simulink model "controller_for_bicycleROS"  (R2021a)
settings: Solver=VariableStepAuto  StartTime=0.0  StopTime=10.0  RelTol=1e-3
values from neighbouring files (symbols this model uses):
  Fyf = zeros(1,57)    [FyfLookUpNewCar.m]    (also in Fyf_loopup_table.mat = [-9372.31873381 -9371.87234491 -9368.75632133 -9360.32413915)
  SlipAngle = -SlipAngle    [FyfLookUpNewCar.m]    (also in Fyf_loopup_table.mat = [0.153111393254 0.147643129209 0.142174865164 0.13670660112 )
  Vx = 15    [controller_setup.m]
libraries: robotlib x22, simulink_extras x1, autolibshared x1, simulink x1
settings Model: Creator=chnwa  LastModifiedBy=chnwa

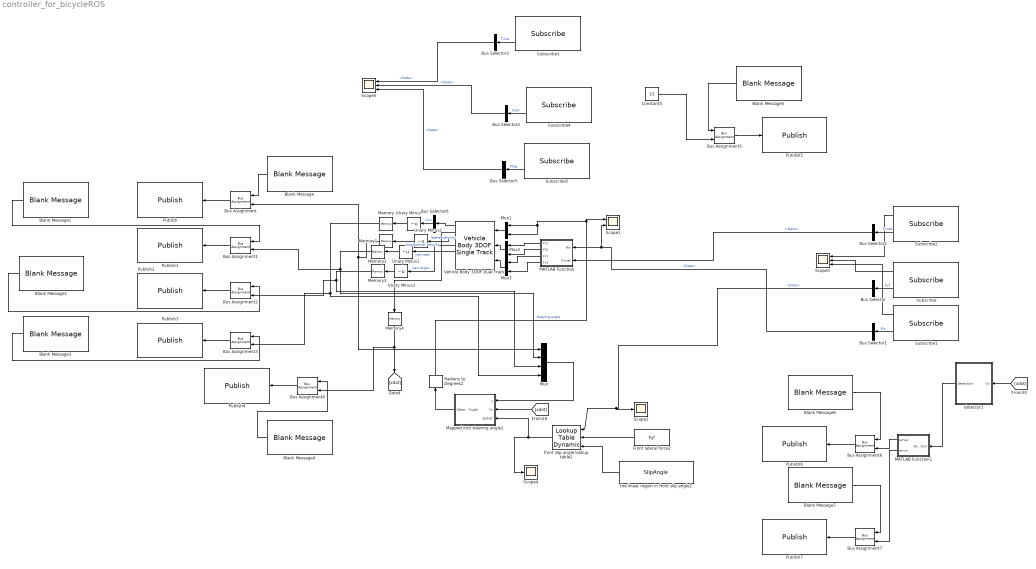
== system controller_for_bicycleROS ==
  Blank Message{,1..7} (8 alike) : robotlib/Blank Message  messageClass=Message  entityType=std_msgs/Float64  messageType=std_msgs/Float64  SampleTime=inf  legacyBusStruct=off
  Bus Assignment{,1..7} (8 alike) : BusAssignment  AssignedSignals=Data
  Bus Selector{,1..5} (6 alike) : BusSelector  OutputSignals=Data
  Bus Selector6 : BusSelector  OutputSignals=InertFrm.Cg.Disp.Y
  Constant5 : Constant  Value=15
  Front lateral force2 : Constant  Value=Fyf
  MATLAB Function : MATLAB Function  TreatAsAtomicUnit=on
  MATLAB Function1 : MATLAB Function  TreatAsAtomicUnit=on
  Mapped into steering angle2 : MATLAB Function  TreatAsAtomicUnit=on
  Memory{,1..3} (4 alike) : Memory
  Memory4 : Memory  InitialCondition=15
  Mux : Mux
  Mux1 : Mux  Inputs=2
  Mux2 : Mux  Inputs=2
  Mux3 : Mux  Inputs=2
  Publish : robotlib/Publish  topicSource=Specify your own  topic=/states1  messageType=std_msgs/Float64  legacyBusStruct=off  messageQueueLength=1
  Publish1 : robotlib/Publish  topicSource=Specify your own  topic=/states2  messageType=std_msgs/Float64  legacyBusStruct=off  messageQueueLength=1
  Publish2 : robotlib/Publish  topicSource=Specify your own  topic=/states3  messageType=std_msgs/Float64  legacyBusStruct=off  messageQueueLength=1
  Publish3 : robotlib/Publish  topicSource=Specify your own  topic=/states4  messageType=std_msgs/Float64  legacyBusStruct=off  messageQueueLength=1
  Publish4 : robotlib/Publish  topicSource=Specify your own  topic=/Vx  messageType=std_msgs/Float64  legacyBusStruct=off  messageQueueLength=1
  Publish5 : robotlib/Publish  topicSource=Specify your own  topic=/Vset  messageType=std_msgs/Float64  legacyBusStruct=off  messageQueueLength=1
  Publish6 : robotlib/Publish  topicSource=Specify your own  topic=/emax  messageType=std_msgs/Float64  legacyBusStruct=off  messageQueueLength=1
  Publish7 : robotlib/Publish  topicSource=Specify your own  topic=/emin  messageType=std_msgs/Float64  legacyBusStruct=off  messageQueueLength=1
  Radians to Degrees2 : simulink_extras/Transformations/Radians to Degrees
  Scope1 : Scope  NumInputPorts=2
  Scope2 : Scope
  Scope3 : Scope  NumInputPorts=3
  Scope4 : Scope
  Scope5 : Scope  NumInputPorts=3
  Subscribe : robotlib/Subscribe  topicSource=Specify your own  topic=/mv1  messageType=std_msgs/Float64  SampleTime=-1  legacyBusStruct=off  messageQueueLength=1
  Subscribe1 : robotlib/Subscribe  topicSource=Specify your own  topic=/mv2  messageType=std_msgs/Float64  SampleTime=-1  legacyBusStruct=off  messageQueueLength=1
  Subscribe2 : robotlib/Subscribe  topicSource=Specify your own  topic=/Fxnet  messageType=std_msgs/Float64  SampleTime=-1  legacyBusStruct=off  messageQueueLength=1
  Subscribe3 : robotlib/Subscribe  topicSource=Specify your own  topic=/Time  messageType=std_msgs/Float64  SampleTime=-1  legacyBusStruct=off  messageQueueLength=1
  Subscribe4 : robotlib/Subscribe  topicSource=Specify your own  topic=/Cost  messageType=std_msgs/Float64  SampleTime=-1  legacyBusStruct=off  messageQueueLength=1
  Subscribe5 : robotlib/Subscribe  topicSource=Specify your own  topic=/Flag  messageType=std_msgs/Float64  SampleTime=-1  legacyBusStruct=off  messageQueueLength=1
  Unary Minus{,1..3} (4 alike) : UnaryMinus
  Vehicle Body 3DOF Dual Track : autolibshared/Vehicle Body 3DOF Single Track  trackMode=Dual  inputMode=External longitudinal forces  frontSteerMode=on  rearSteerMode=off  windMode=off  muMode=off  extFMode=off  extMMode=off  htchFMode=off  htchMMode=off  extXo=off  extpsio=off  extxdoto=off  extro=off  extYo=off  extTamb=off  extydoto=off  aMode=2  NF=2  NR=2  m=2272  a=1.11  b=1.67  h=0.35  dh=1  hh=0.2  X_o=0  xdot_o=15  CalphaMode=off  sigmaMode=on  d=0  hl=0  w=[1.4,1.4]  Cy_f=1.822e5  Cy_r=1.822e5  sigma_f=.1  sigma_r=.1  alpha_f_brk=[-.1 .1]  Cy_f_data=[-9e3 9e3]  alpha_r_brk=[-.1 .1]  Cy_r_data=[-9e3 9e3]  Y_o=0  ydot_o=0  Izz=4600  psi_o=0  r_o=0  Af=2  Cd=.3  Cl=.1  Cpm=.1  beta_w=[0:0.01:0.3]  Cs=[0:0.03:0.9]  Cym=[0:0.01:0.3]  Pabs=101325  Tair=273  g=9.81  mu=0.7  xdot_tol=.01  Fznom=5000  Fxtire_sat=7e4  Fytire_sat=7e4  longOff=0  latOff=0  vertOff=0  wrapAng=off
      settings: SourceProductBaseCode=PW,DR,MT,UV,VE
  detector1 : Subsystem
  front slip angle lookup table2 : simulink/Lookup Tables/Lookup Table Dynamic  LookUpMeth=Interpolation-Use End Values  OutDataType=fixdt('double')  OutScaling=[]  OutputDataTypeScalingMode=Specify via dialog  OutDataTypeStr=double  DoSatur=off
  tire linear region in front slip angle2 : Constant  Value=SlipAngle
  wires:
  MATLAB Function/2(Fl2) -> Mux2/2
  Mapped into steering angle2/1(SteeringAngle) -> Radians to Degrees2/1
  Bus Selector4/1 -> Scope5/2  "<Data>"
  Constant5/1 -> Bus Assignment5/2
  Bus Assignment4/1 -> Publish4/1
  Bus Selector5/1 -> Scope5/3  "<Data>"
  Bus Selector3/1 -> Scope5/1  "<Data>"
  Vehicle Body 3DOF Dual Track/3 -> Unary Minus2/1  "lateral velocity"
  Bus Selector/1 -> Scope2/1, front slip angle lookup table2/1  "<Data>"
  Front lateral force2/1 -> front slip angle lookup table2/2
  detector1/1(detection) -> MATLAB Function1/1(detection)
  Blank Message2/1 -> Bus Assignment2/1
  Subscribe/2 -> Bus Selector/1  "Fyf"
  Bus Assignment7/1 -> Publish7/1
  Blank Message1/1 -> Bus Assignment1/1
  MATLAB Function/3(Fr1) -> Mux3/1
  Blank Message7/1 -> Bus Assignment7/1
  Blank Message6/1 -> Bus Assignment6/1
  Bus Assignment3/1 -> Publish3/1
  Bus Selector1/1 -> Scope1/2, MATLAB Function/1(Mx)  "<Data>"
  Subscribe5/2 -> Bus Selector5/1  "Flag"
  Bus Assignment2/1 -> Publish2/1
  Bus Assignment6/1 -> Publish6/1
  Vehicle Body 3DOF Dual Track/4 -> Unary Minus3/1  "yaw angle"
  Subscribe1/2 -> Bus Selector1/1  "Mx"
  Bus Assignment/1 -> Publish/1
  MATLAB Function1/1(emax) -> Bus Assignment6/2
  Bus Selector2/1 -> MATLAB Function/2(Fxnet)  "<Data>"
  Subscribe/1 -> Scope3/2
  Blank Message/1 -> Bus Assignment/1
  Subscribe1/1 -> Scope3/3
  Blank Message4/1 -> Bus Assignment4/1
  Radians to Degrees2/1 -> Mux1/2, Mux1/1, Scope1/1  "steering angle"
  Subscribe4/2 -> Bus Selector4/1  "Cost"
  Bus Assignment5/1 -> Publish5/1
  Subscribe3/2 -> Bus Selector3/1  "Time"
  front slip angle lookup table2/1 -> Scope4/1, Mapped into steering angle2/3(alphaf)
  MATLAB Function1/2(emin) -> Bus Assignment7/2
  MATLAB Function/4(Fr2) -> Mux3/2
  Bus Selector6/1 -> Unary Minus/1  "<Y>"
  MATLAB Function/1(Fl1) -> Mux2/1
  Blank Message5/1 -> Bus Assignment5/1
  Mux/1 -> Mapped into steering angle2/1(x)
  Bus Assignment1/1 -> Publish1/1
  Subscribe2/2 -> Bus Selector2/1  "Fxnet"
  Vehicle Body 3DOF Dual Track/5 -> Unary Minus1/1  "yaw rate"
  Blank Message3/1 -> Bus Assignment3/1
  Subscribe2/1 -> Scope3/1
  tire linear region in front slip angle2/1 -> front slip angle lookup table2/3
  [xdot] -> Mapped into steering angle2/2(Vx)
  [xdot] -> detector1/1(Vx)
  Vehicle Body 3DOF Dual Track/2 -> Memory4/1  "longitudinal velocity"
  Mux2/1 -> Vehicle Body 3DOF Dual Track/2
  Mux1/1 -> Vehicle Body 3DOF Dual Track/1
  Mux3/1 -> Vehicle Body 3DOF Dual Track/3
  Vehicle Body 3DOF Dual Track/1 -> Bus Selector6/1
  Unary Minus/1 -> Memory/1
  Unary Minus2/1 -> Memory1/1
  Unary Minus3/1 -> Memory3/1
  Unary Minus1/1 -> Memory2/1
  Memory/1 -> Mux/4, Bus Assignment3/2
  Memory1/1 -> Bus Assignment/2, Mux/1
  Memory2/1 -> Mux/2, Bus Assignment1/2
  Memory3/1 -> Mux/3, Bus Assignment2/2
  Memory4/1 -> [xdot], Bus Assignment4/2

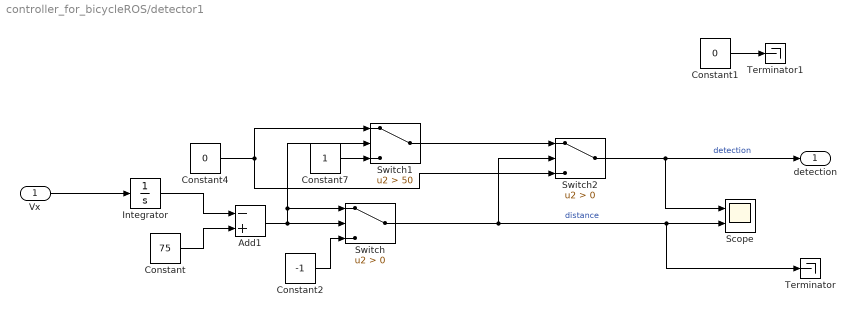
== system controller_for_bicycleROS/detector1 ==
  Vx : Inport
  Add1 : Sum  Inputs=-+
  Constant : Constant  Value=75
  Constant1 : Constant  Value=0
  Constant2 : Constant  Value=-1
  Constant4 : Constant  Value=0
  Constant7 : Constant
  Integrator : Integrator
  Scope : Scope  NumInputPorts=2
  Switch : Switch  Criteria=u2 > Threshold
  Switch1 : Switch  Criteria=u2 > Threshold  Threshold=50
  Switch2 : Switch  Criteria=u2 > Threshold
  Terminator : Terminator
  Terminator1 : Terminator
  detection : Outport
  wires:
  Constant2/1 -> Switch/3
  Constant4/1 -> Switch2/3, Switch1/1
  Vx/1 -> Integrator/1
  Integrator/1 -> Add1/1
  Switch/1 -> Switch2/2, Terminator/1, Scope/2  "distance"
  Constant7/1 -> Switch1/3
  Add1/1 -> Switch1/2, Switch/1, Switch/2
  Switch1/1 -> Switch2/1
  Constant/1 -> Add1/2
  Switch2/1 -> detection/1, Scope/1  "detection"
  Constant1/1 -> Terminator1/1

== matlab function controller_for_bicycleROS/MATLAB Function1 ==
  data: detection input; emax output; emin output
function [emax,emin] = fcn(detection)

if detection
    emax=6;
    emin=4;
else
    emax=10;
    emin=-10;
end

== matlab function controller_for_bicycleROS/Mapped into steering angle2 ==
  data: x input; Vx input; alphaf input; SteeringAngle output
function SteeringAngle = fcn(x,Vx, alphaf)

lf = 1.11;  % distance from front axle to the mass center

Vy = x(1); %lateral velocity
r = x(2);  %yaw rate
SteeringAngle = Vy/Vx+lf*r/Vx-alphaf;

== matlab function controller_for_bicycleROS/MATLAB Function ==
  data: Fl1 output; Mx input; Fl2 output; Fxnet input; Fr1 output; Fr2 output
function [Fl1,Fl2,Fr1,Fr2] = fcn(Mx,Fxnet)

w = 1.875; % the width of the car

Fwf = zeros(2,1);
Fwr = zeros(2,1);

if Mx > 0
    Fwf(1) = Fxnet/2+0;
    Fwf(2) = Fxnet/2-Mx/w;
    Fwr(1) = 0;
    Fwr(2) = -Mx/w;
elseif Mx < 0
    Fwf(1) = Fxnet/2+Mx/w;
    Fwf(2) = Fxnet/2+0;
    Fwr(1) = Mx/w;
    Fwr(2) = 0;
else
    Fwf(1) = Fxnet/2+0;
    Fwf(2) = Fxnet/2+0;
    Fwr(1) = 0;
    Fwr(2) = 0;
end
Fl1 = Fwf(1);
Fl2 = Fwr(1);
Fr1 = Fwf(2);
Fr2 = Fwr(2);
